simulink model "RobotController21"  (R2017a)
settings: Solver=VariableStepAuto  StartTime=0.0  StopTime=500.0  RelTol=1e-3
settings Model: Creator=Carapinha  LastModifiedBy=Carapinha

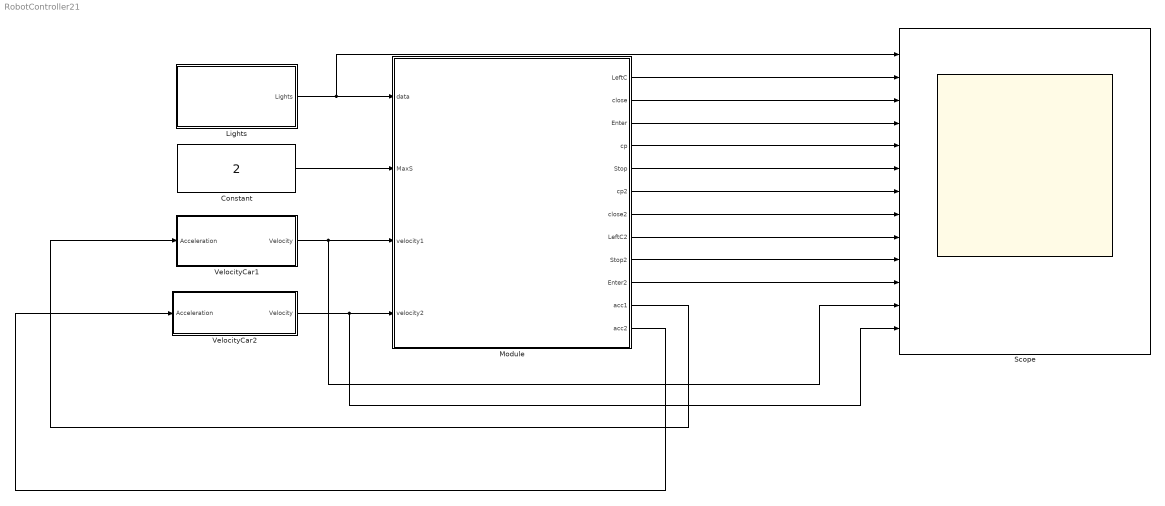
== system RobotController21 ==
  Constant : Constant  Value=2
  Lights : Stateflow chart  TreatAsAtomicUnit=on
  Module : Stateflow chart  TreatAsAtomicUnit=on
  Scope : Scope  NumInputPorts=13
  VelocityCar1 : Subsystem
  VelocityCar2 : Subsystem
  wires:
  Module/7(close2) -> Scope/8
  Module/4(cp) -> Scope/5
  Module/6(cp2) -> Scope/7
  Module/5(Stop) -> Scope/6
  Module/10(Enter2) -> Scope/11
  Module/1(LeftC) -> Scope/2
  Module/2(close) -> Scope/3
  Constant/1 -> Module/2(MaxS)
  Module/9(Stop2) -> Scope/10
  Module/8(LeftC2) -> Scope/9
  Lights/1(Lights) -> Scope/1, Module/1(data)
  Module/3(Enter) -> Scope/4
  Module/11(acc1) -> VelocityCar1/1("Acceleration ")
  Module/12(acc2) -> VelocityCar2/1(Acceleration)
  VelocityCar1/1(Velocity) -> Scope/12, Module/3(velocity1)
  VelocityCar2/1(Velocity) -> Scope/13, Module/4(velocity2)

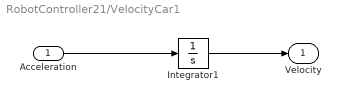
== system RobotController21/VelocityCar1 ==
  "Acceleration " : Inport
  Integrator1 : Integrator  InitialCondition=1
  Velocity : Outport
  wires:
  "Acceleration "/1 -> Integrator1/1
  Integrator1/1 -> Velocity/1

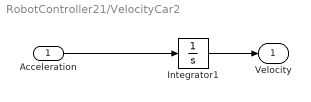
== system RobotController21/VelocityCar2 ==
  Acceleration : Inport
  Integrator1 : Integrator  InitialCondition=1
  Velocity : Outport
  wires:
  Acceleration/1 -> Integrator1/1
  Integrator1/1 -> Velocity/1

== stateflow chart RobotController21/Lights ==
  state Red
    entry:
    Lights = 0;
  state Green
    entry:
    Lights = 1;
  (default) -> Red
  Green -> Red : [after(0.7, sec)]
  Red -> Green : [after(0.7,sec)]
  data: Lights output

== stateflow chart RobotController21/Module ==
  state Main
    state Robot1 [parallel]
      settings: executionOrder=1
      state move3
        entry:
        LeftC = 0;
        close = 0;
        Enter = 1;
        cp = 0;
        Stop = 0;
        acc1 = 0;
      state move1
        entry:
        LeftC = 1;
        close = 0;
        Enter = 0;
        cp = 0;
        Stop = 0;
      state move2
        entry:
        LeftC = 0;
        close = 1;
        Enter = 0;
        cp = 0;
        Stop = 0;
      state Accel
        entry:
        LeftC = 0;
        close = 0;
        Enter = 1;
        cp = 0;
        Stop = 0;
        acc1 = 0.01;
      state Decel
        entry:
        LeftC = 0;
        close = 0;
        Enter = 0;
        cp = 1;
        Stop = 0;
        acc1 = -0.01;
      state Wait
        entry:
        LeftC = 0;
        close = 0;
        Enter = 0;
        cp = 0;
        Stop = 1;
        acc1 = 0;
      Main.Robot1.move3 -> Main.Robot1.move1 : [after(0.3,sec)]
      (default) -> Main.Robot1.move1
      Main.Robot1.move1 -> Main.Robot1.move2 : [after(0.3,sec)]
      Main.Robot1.move2 -> Main.Robot1.move3 [order 1] : [Permission1 == 1]
      Main.Robot1.move2 -> Main.Robot1.Decel [order 2] : [after(0.3,sec)]
      Main.Robot1.Accel -> Main.Robot1.move3 : [velocity1 >= MaxS]
      Main.Robot1.Decel -> Main.Robot1.Accel [order 1] : [Permission1 == 1]
      Main.Robot1.Decel -> Main.Robot1.Wait [order 2] : [velocity1 <= 0]
      Main.Robot1.Wait -> Main.Robot1.Accel [order 1] : [Permission1 == 1]
      Main.Robot1.Wait -> Main.Robot1.Wait [order 2] : [Permission1 == 0]
    state Robot2 [parallel]
      settings: executionOrder=3
      state move3
        entry:
        LeftC2 = 0;
        close2 = 0;
        Enter2 = 1;
        cp2 = 0;
        Stop2 = 0;
        acc2 = 0;
      state move1
        entry:
        LeftC2 = 1;
        close2 = 0;
        Enter2 = 0;
        cp2 = 0;
        Stop2 = 0;
      state move2
        entry:
        LeftC2 = 0;
        close2 = 1;
        Enter2 = 0;
        cp2 = 0;
        Stop2 = 0;
      state Accel
        entry:
        LeftC2 = 0;
        close2 = 0;
        Enter2 = 1;
        cp2 = 0;
        Stop2 = 0;
        acc2 = 0.01;
      state Decel
        entry:
        LeftC2 = 0;
        close2 = 0;
        Enter2 = 0;
        cp2 = 1;
        Stop2 = 0;
        acc2 = -0.01;
      state Wait
        entry:
        LeftC2 = 0;
        close2 = 0;
        Enter2 = 0;
        cp2 = 0;
        Stop2 = 1;
        acc2 = 0;
      Main.Robot2.move3 -> Main.Robot2.move1 : [after(0.3,sec)]
      (default) -> Main.Robot2.move1
      Main.Robot2.move1 -> Main.Robot2.move2 : [after(0.3,sec)]
      Main.Robot2.move2 -> Main.Robot2.move3 [order 1] : [Permission2 == 1]
      Main.Robot2.move2 -> Main.Robot2.Decel [order 2] : [after(0.3,sec)]
      Main.Robot2.Accel -> Main.Robot2.move3 : [velocity2 >= MaxS]
      Main.Robot2.Decel -> Main.Robot2.Accel [order 1] : [Permission2 == 1]
      Main.Robot2.Decel -> Main.Robot2.Wait [order 2] : [velocity2 <= 0]
      Main.Robot2.Wait -> Main.Robot2.Accel [order 1] : [Permission2 == 1]
      Main.Robot2.Wait -> Main.Robot2.Wait [order 2] : [Permission2 == 0]
    state Controller [parallel]
      settings: executionOrder=2
      state Green
        entry:
        Permission1 = 1;
        Permission2 = 0;
      state RobotState
      state RobotState3
      state Red
        entry:
        Permission1 = 0;
        Permission2 = 1;
      RobotState3 -> RobotState : [LeftC == 1 || LeftC2 == 1]
      (default) -> RobotState
      (junction 79) -> Green [order 1] : [data == 1 && Enter2 ~= 1]
      Green -> RobotState3
      RobotState -> (junction 79) : [(close == 1 || Stop == 1) || (close2 == 1 || Stop2 == 1)]
      (junction 79) -> Red [order 2] : [data == 0 && Enter ~= 1]
      Red -> RobotState3
  (default) -> Main
  data: data input; LeftC output; close output; Enter output; cp output; Stop output; MaxS input; cp2 output; Permission1 local; Permission2 local; close2 output; LeftC2 output; Stop2 output; Enter2 output; Decel local; Accel local; acc1 output; acc2 output; velocity1 input; velocity2 input
